simulink model "Block_DT"  (R2022a)
settings: Solver=ode23tb  StartTime=0.0  StopTime=5  MaxStep=1e-4  RelTol=1e-5
undefined symbols (not defined in the file): DT
libraries: dspsigattribs x1, dspstat3 x1
settings Model: Creator=админ  LastModifiedBy=админ

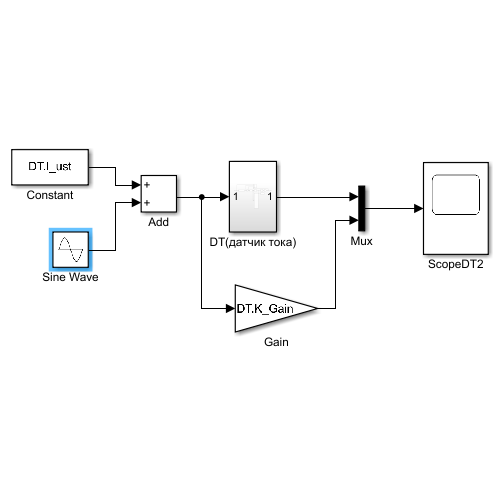
[thumbnail: Simulink's stored preview of the top-level diagram]
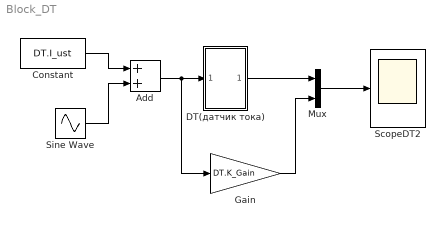
== system Block_DT ==
  Add : Sum
  Constant : Constant  Value=DT.I_ust
  DT(датчик тока) : Subsystem
  Gain : Gain  Gain=DT.K_Gain
  Mux : Mux  Inputs=2
  ScopeDT2 : Scope
  Sine Wave : Sin  Amplitude=DT.Sine_Wave.amplitude  Frequency=DT.Sine_Wave.freq  SampleTime=0
  wires:
  Constant/1 -> Add/1
  Sine Wave/1 -> Add/2
  Add/1 -> Gain/1, DT(датчик тока)/1(In1)
  DT(датчик тока)/1(Out1) -> Mux/1
  Gain/1 -> Mux/2
  Mux/1 -> ScopeDT2/1

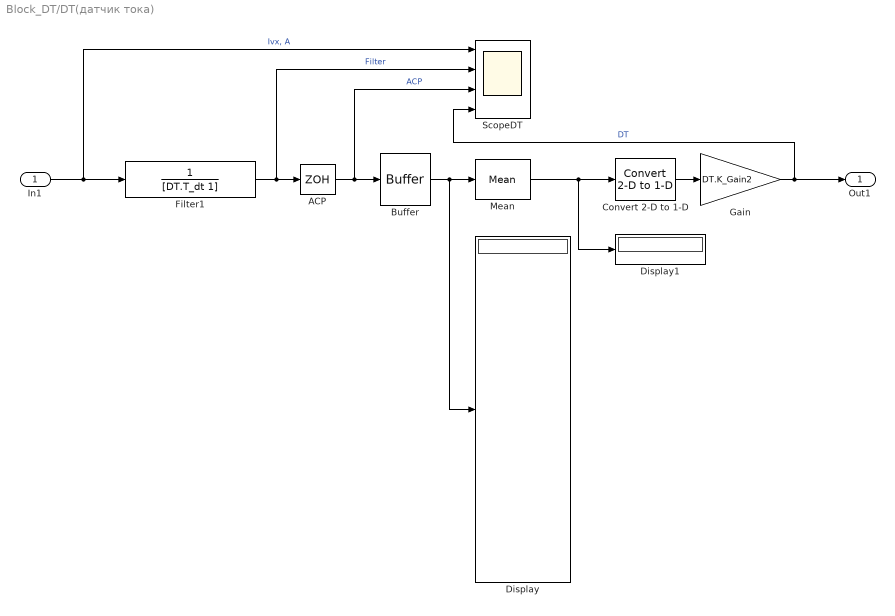
== system Block_DT/DT(датчик тока) ==
  In1 : Inport
  Buffer : Buffer  N=DT.Buffer_size  OutputFrames=off
  Convert 2-D to 1-D : dspsigattribs/Convert 2-D to 1-D
      settings: SourceProductBaseCode=DS
  Display : Display
  Display1 : Display
  Filter1 : TransferFcn  Denominator=[DT.T_dt 1]
  Gain : Gain  Gain=DT.K_Gain2
  Mean : dspstat3/Mean  run=off  InputProcessing=Columns as channels (frame based)  reset_popup=None  directionMode=Each column  dimension=1  roiEnable=off  roiType=Rectangles  roiPortion=Entire ROI  roiOutput=Individual statistics for each ROI  roiFlag=off  roundingMode=Floor  overflowMode=off  outputDataTypeStr=Inherit: Same as accumulator  outputMin=[]  outputMax=[]  outputLastDataTypeStr=Inherit: Same as accumulator
  ScopeDT : Scope  NumInputPorts=4
  АСР : ZeroOrderHold  SampleTime=DT.T_kv1
  Out1 : Outport
  wires:
  Filter1/1 -> ScopeDT/2, АСР/1  "Filter"
  АСР/1 -> ScopeDT/3, Buffer/1  "АСР"
  Buffer/1 -> Display/1, Mean/1
  Gain/1 -> Out1/1, ScopeDT/4  "DT"
  Mean/1 -> Convert 2-D to 1-D/1, Display1/1
  In1/1 -> Filter1/1, ScopeDT/1  "Ivx, А"
  Convert 2-D to 1-D/1 -> Gain/1
